simulink model "test_comp"  (R2024a)
settings: Solver=VariableStepAuto  StartTime=0.0  StopTime=10.0  RelTol=1e-3
libraries: simulink x1
settings Model: Creator=storm  LastModifiedBy=storm

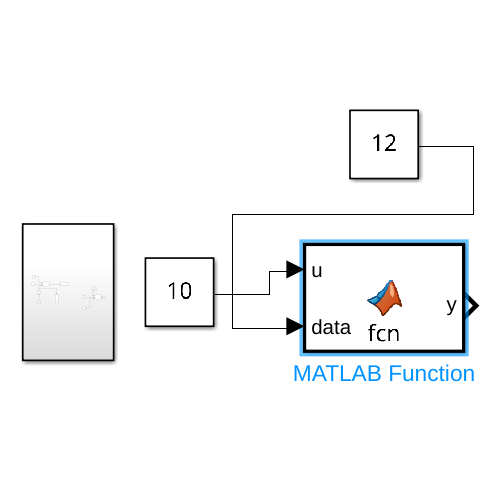
[thumbnail: Simulink's stored preview of the top-level diagram]
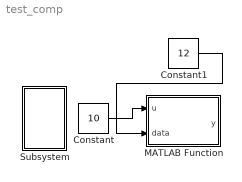
== system test_comp ==
  Constant : Constant  Value=10
  Constant1 : Constant  Value=12
  MATLAB Function : MATLAB Function  TreatAsAtomicUnit=on
  Subsystem : Subsystem
  wires:
  Constant/1 -> MATLAB Function/1(u)
  Constant1/1 -> MATLAB Function/2(data)

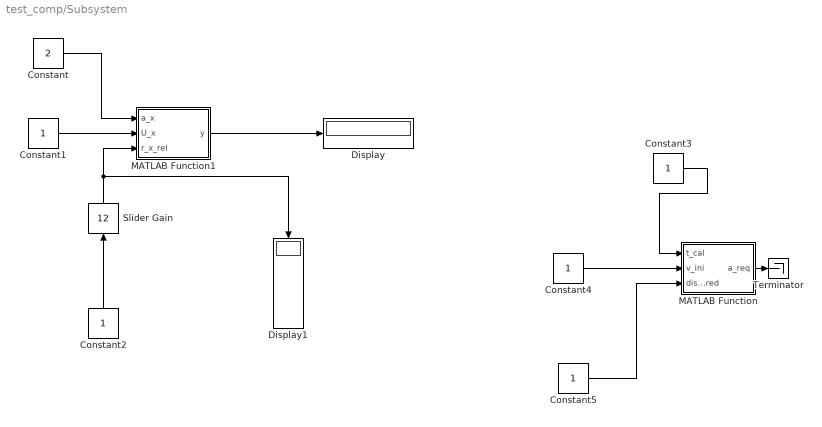
== system test_comp/Subsystem ==
  Constant : Constant  Value=2
  Constant{1..5} (5 alike) : Constant
  Display : Display
  Display1 : Display
  MATLAB Function : MATLAB Function  TreatAsAtomicUnit=on
  MATLAB Function1 : MATLAB Function  TreatAsAtomicUnit=on
  Slider Gain : simulink/Math Operations/Slider Gain  gain=12  low=0  high=110
  Terminator : Terminator
  wires:
  MATLAB Function1/1(y) -> Display/1
  Constant5/1 -> MATLAB Function/3(dist_covered)
  Constant1/1 -> MATLAB Function1/2(U_x)
  Constant3/1 -> MATLAB Function/1(t_cal)
  MATLAB Function/1(a_req) -> Terminator/1
  Constant4/1 -> MATLAB Function/2(v_ini)
  Constant/1 -> MATLAB Function1/1(a_x)
  Slider Gain/1 -> MATLAB Function1/3(r_x_rel), Display1/1
  Constant2/1 -> Slider Gain/1

== matlab function test_comp/Subsystem/MATLAB Function1 ==
  data: a_x input; y output; U_x input; r_x_rel input
function y = fcn(a_x, U_x, r_x_rel)
    eq1 = [0.5*a_x, U_x, -r_x_rel];
    r = roots(eq1);
    y = r(2);
    
end

== matlab function test_comp/Subsystem/MATLAB Function ==
  data: t_cal input; a_req output; v_ini input; dist_covered input
function a_req = fcn(t_cal, v_ini, dist_covered)
    a_req = (2/(t_cal^2))*(dist_covered - (v_ini*t_cal));
end

== matlab function test_comp/MATLAB Function ==
  data: u input; y output; data input
function y = fcn(u, data)

y = u- data;
